simulink model "mdlref_conversion"  (Simulink 6.0)
settings: Solver=ode5  StartTime=0.0  StopTime=30  RelTol=1e-3
settings Model: Creator=The MathWorks Inc.  LastModifiedBy=batserve  ExtModeAutoUpdateStatusClock=off  ProdHWDeviceType=Specified
settings DataIOCC: SignalLoggingName=logsOut
settings OptimizationCC: InlineParams=on
settings DebuggingCC: CheckExecutionContextPreStartOutputMsg=on  CheckExecutionContextRuntimeOutputMsg=on  SolverPrmCheckMsg=none
settings HardwareCC: ProdHWDeviceType=Specified  TargetHWDeviceType=32-bit Generic  ProdEqTarget=off
settings ModelReferenceCC: UpdateModelReferenceTargets=IfOutOfDate
settings RTWCC: ProcessScript=grt_make_rtw_hook

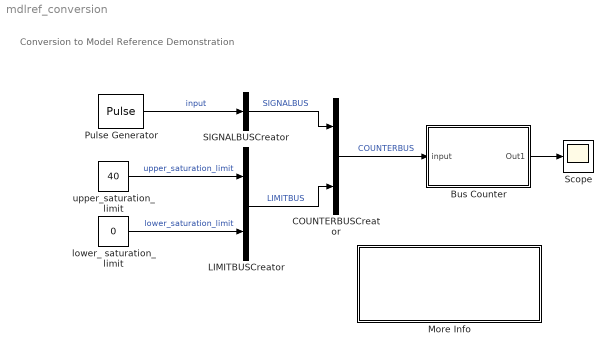
== system mdlref_conversion ==
  note: Conversion to Model Reference Demonstration
  Bus Counter : Subsystem  TreatAsAtomicUnit=on  PropExecContextAcrossSSBoundary=on
  COUNTERBUSCreator : BusCreator  DialogController=Simulink.DDGSource_Bus  Inputs=2
  LIMITBUSCreator : BusCreator  DialogController=Simulink.DDGSource_Bus  Inputs=2
  More Info : Subsystem  PropExecContextAcrossSSBoundary=on
      settings: OpenFcn=mdlref_conversionscript
      mask Display: disp('Double click here \nfor a step-by-step\ntutorial on this model')
  Pulse Generator : DiscretePulseGenerator  Amplitude=int32(1)  SampleTime=0.1
  SIGNALBUSCreator : BusCreator  DialogController=Simulink.DDGSource_Bus  Inputs=1
  Scope : Scope
      settings: TimeRange=30  YMax=50  DataFormat=Array
  lower_ saturation_ limit : Constant  Value=0  OutDataTypeMode=int32  SampleTime=0.1
  upper_saturation_limit : Constant  Value=40  OutDataTypeMode=int32  SampleTime=0.1
  wires:
  upper_saturation_limit/1 -> LIMITBUSCreator/1  "upper_saturation_limit"
  lower_ saturation_ limit/1 -> LIMITBUSCreator/2  "lower_saturation_limit"
  LIMITBUSCreator/1 -> COUNTERBUSCreator/2  "LIMITBUS"
  Pulse Generator/1 -> SIGNALBUSCreator/1  "input"
  COUNTERBUSCreator/1 -> Bus Counter/1(" input")  "COUNTERBUS"
  Bus Counter/1(Out1) -> Scope/1
  SIGNALBUSCreator/1 -> COUNTERBUSCreator/1  "SIGNALBUS"

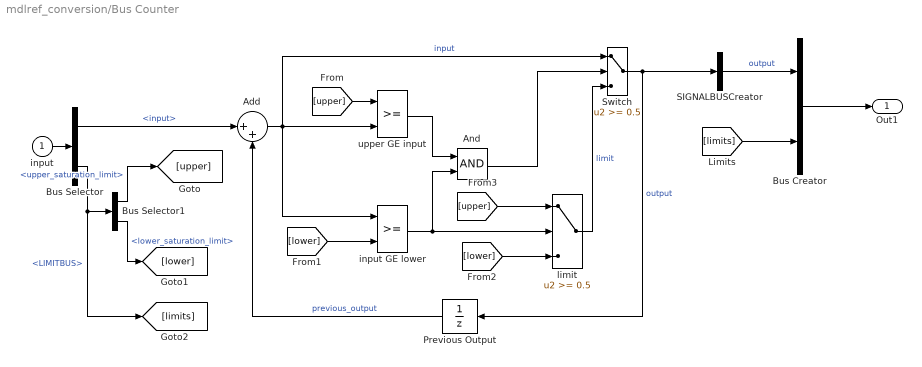
== system mdlref_conversion/Bus Counter ==
  " input" : Inport  Port=1  LatchInput=off
  " input GE lower" : RelationalOperator  Priority=1  InputSameDT=on
      settings: AttributesFormatString=\n
  " limit" : Switch  Threshold=0.5  SaturateOnIntegerOverflow=on  InputSameDT=on
  Add : Sum  Inputs=|++  OutScaling=2^-10
  And : Logic
  Bus Creator : BusCreator  DialogController=Simulink.DDGSource_Bus  Inputs=2
  Bus Selector : BusSelector  DialogController=Simulink.DDGSource_Bus  OutputSignals=SIGNALBUS.input,LIMITBUS
  Bus Selector1 : BusSelector  DialogController=Simulink.DDGSource_Bus  OutputSignals=upper_saturation_limit,lower_saturation_limit
  Previous Output : UnitDelay  Orientation=left  SampleTime=-1
  SIGNALBUSCreator : BusCreator  DialogController=Simulink.DDGSource_Bus  Inputs=1
  Switch : Switch  Threshold=0.5  SaturateOnIntegerOverflow=on  InputSameDT=on
  upper GE input : RelationalOperator  Priority=0  InputSameDT=on
      settings: AttributesFormatString=\n
  Out1 : Outport
  wires:
  [upper] -> " limit"/1
  Switch/1 -> SIGNALBUSCreator/1, Previous Output/1  "output"
  " limit"/1 -> Switch/3  "limit"
  upper GE input/1 -> And/1
  Previous Output/1 -> Add/2  "previous_output"
  [lower] -> " limit"/3
  [upper] -> upper GE input/1
  [lower] -> " input GE lower"/2
  " input GE lower"/1 -> " limit"/2, And/2
  And/1 -> Switch/2
  Add/1 -> Switch/1, upper GE input/2, " input GE lower"/1  "input"
  " input"/1 -> Bus Selector/1
  Bus Selector/2 -> [limits], Bus Selector1/1  "<LIMITBUS>"
  Bus Selector/1 -> Add/1  "<input>"
  Bus Selector1/1 -> [upper]  "<upper_saturation_limit>"
  Bus Selector1/2 -> [lower]  "<lower_saturation_limit>"
  Bus Creator/1 -> Out1/1
  [limits] -> Bus Creator/2
  SIGNALBUSCreator/1 -> Bus Creator/1  "output"

== system mdlref_conversion/More Info ==
  note: This demonstration shows how signals may be grouped and ungrouped while
      | retaining their names.  In this demonstration, 5 signals are created and labelled
      | appropriately.  These signals are then mux'd together to create a bus of signals.
      | This bus of signals is then fed into the Bus Selector block.  Inside of the Bus
      | Selector block, the Pulse and Chirp signals are chosen to be output from the
      | original signal bus.
      |
      | It is possible to place a nest signal buses and then still retrieve the original signal
      | with its label.
  note: Bus Block Demonstration
